simulink model "sim_instalacja_grzejnikowa_modele_Tkz"  (R2021b)
settings: Solver=VariableStepAuto  StartTime=0.0  StopTime=10.0  MaxStep=5  RelTol=1e-3
undefined symbols (not defined in the file): dspr, k, skok_czas, T0_dwupunkt, T0_klasyczna, T_dwupunkt, T_klasyczna
settings Model: Creator=adams  LastModifiedBy=adams

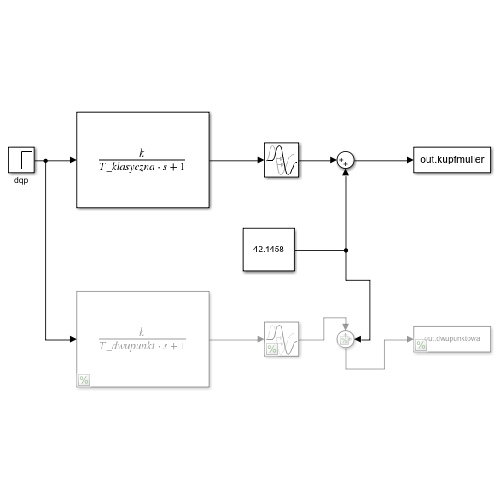
[thumbnail: Simulink's stored preview of the top-level diagram]
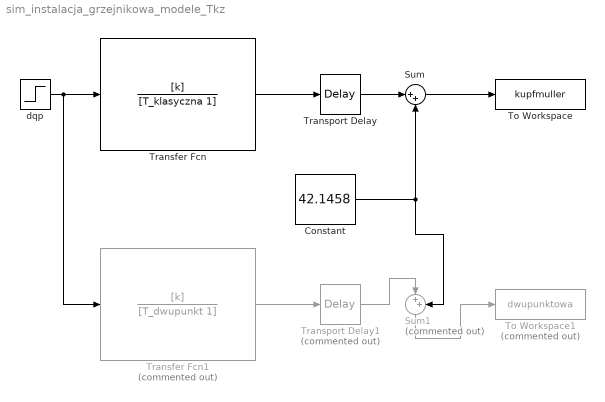
== system sim_instalacja_grzejnikowa_modele_Tkz ==
  Constant : Constant  Value=42.1458
  Sum : Sum  Inputs=|++
  Sum1 : Sum  Commented=on  Inputs=|++
  To Workspace : ToWorkspace  VariableName=kupfmuller  SampleTime=-1
  To Workspace1 : ToWorkspace  Commented=on  VariableName=dwupunktowa  SampleTime=-1
  Transfer Fcn : TransferFcn  Numerator=[k]  Denominator=[T_klasyczna 1]
  Transfer Fcn1 : TransferFcn  Commented=on  Numerator=[k]  Denominator=[T_dwupunkt 1]
  Transport Delay : TransportDelay  DelayTime=T0_klasyczna  BufferSize=32768
  Transport Delay1 : TransportDelay  Commented=on  DelayTime=T0_dwupunkt  BufferSize=32768
  dqp : Step  Time=skok_czas  After=dspr  SampleTime=0
  wires:
  Sum1/1 -> To Workspace1/1
  Transfer Fcn/1 -> Transport Delay/1
  Sum/1 -> To Workspace/1
  Transport Delay/1 -> Sum/1
  Transfer Fcn1/1 -> Transport Delay1/1
  Transport Delay1/1 -> Sum1/1
  dqp/1 -> Transfer Fcn1/1, Transfer Fcn/1
  Constant/1 -> Sum/2, Sum1/2
